simulink model "controller_angular_rate_roll"  (R2020a)
settings: Solver=FixedStepAuto  StartTime=0.0  StopTime=10.0  FixedStep=1/sim_freq  RelTol=1e-3
undefined symbols (not defined in the file): body_rates_dterm_cutoff, body_rates_filter_denom, body_rates_filter_num, d, DiscIntNeverNeededParam, Ixx, K_pd, K_pi, K_pp, max_T, p_int_lim, p_max, tau_T
libraries: simulink x2
settings Model: Creator=francois  LastModifiedBy=murray

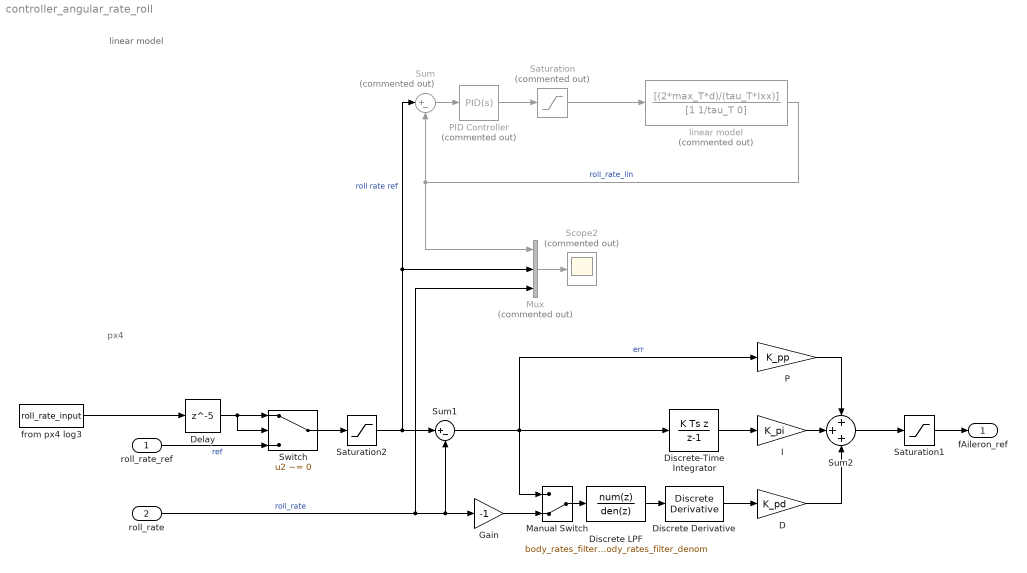
== system controller_angular_rate_roll ==
  note: px4
  note: linear model
  roll_rate_ref : Inport
  roll_rate : Inport  Port=2
  D : Gain  Gain=K_pd
  Delay : Delay  DelayLength=5
  Discrete Derivative : simulink/Discrete/Discrete Derivative  gainval=1.0  ICPrevScaledInput=0.0  OutMin=[]  OutMax=[]  OutDataType=fixdt(1, 16)  OutScaling=2^-10  DoSatur=off
  Discrete LPF : DiscreteTransferFcn  Numerator=body_rates_filter_num  Denominator=body_rates_filter_denom
  Discrete-Time Integrator : DiscreteIntegrator  IntegratorMethod=Integration: Backward Euler  SampleTime=-1  LimitOutput=on  UpperSaturationLimit=p_int_lim  LowerSaturationLimit=-p_int_lim  ICPrevOutput=DiscIntNeverNeededParam  ICPrevScaledInput=DiscIntNeverNeededParam
  Gain : Gain  Gain=-1
  I : Gain  Gain=K_pi
  Manual Switch : ManualSwitch  CurrentSetting=0
  Mux : Mux  Commented=on  Inputs=3
  P : Gain  Gain=K_pp
  "PID Controller " : simulink/Continuous/PID Controller  Commented=on  Controller=PID  Form=Parallel  TimeDomain=Continuous-time  UseExternalTs=off  SampleTime=-1  IntegratorMethod=Forward Euler  FilterMethod=Forward Euler  ControllerParametersSource=internal  P=K_pp  I=K_pi  D=K_pd  UseFilter=on  N=body_rates_dterm_cutoff*10  TunerSelectOption=Transfer Function Based (PID Tuner App)  InitialConditionSource=internal  InitialConditionForIntegrator=0  InitialConditionForFilter=0  DifferentiatorICPrevScaledInput=0  ExternalReset=none  TrackingMode=off  Kt=1  LimitOutput=off  UpperSaturationLimit=inf  LowerSaturationLimit=-inf  LinearizeAsGain=on  AntiWindupMode=none  Kb=1  POutMin=[]  POutMax=[]  IOutMin=[]  IOutMax=[]  DOutMin=[]  DOutMax=[]  NOutMin=[]  NOutMax=[]  SumOutMin=[]  SumOutMax=[]  SaturationOutMin=[]  SaturationOutMax=[]  PParamMin=[]  PParamMax=[]  IParamMin=[]  IParamMax=[]  DParamMin=[]  DParamMax=[]  NParamMin=[]  NParamMax=[]  KbParamMin=[]  KbParamMax=[]  KtParamMin=[]  KtParamMax=[]  KbOutMin=[]  KbOutMax=[]  KtOutMin=[]  KtOutMax=[]  IntegratorOutMin=[]  IntegratorOutMax=[]  FilterOutMin=[]  FilterOutMax=[]  SumI1OutMin=[]  SumI1OutMax=[]  SumI2OutMin=[]  SumI2OutMax=[]  SumI3OutMin=[]  SumI3OutMax=[]  SumI4OutMin=[]  SumI4OutMax=[]  SumDOutMin=[]  SumDOutMax=[]  DifferentiatorOutMin=[]  DifferentiatorOutMax=[]  FilterDiffOutCoefMin=[]  FilterDiffOutCoefMax=[]  ReciprocalOutMin=[]  ReciprocalOutMax=[]  SumDenOutMin=[]  SumDenOutMax=[]  SumNumOutMin=[]  SumNumOutMax=[]  DivideOutMin=[]  DivideOutMax=[]  UdiffTsProdOutMin=[]  UdiffTsProdOutMax=[]  NTsProdOutMin=[]  NTsProdOutMax=[]  UintegralTsProdOutMin=[]  UintegralTsProdOutMax=[]  UngainTsProdOutMin=[]  UngainTsProdOutMax=[]  IntegratorContinuousStateAttributes=''  IntegratorStateMustResolveToSignalObject=off  IntegratorRTWStateStorageClass=Auto  FilterContinuousStateAttributes=''  FilterStateMustResolveToSignalObject=off  FilterRTWStateStorageClass=Auto  ParallelPVariant=InternalParameters  IdealPVariant=Disabled  IVariant=InternalParameters  DVariant=InternalParameters  IntegratorVariant=Continuous  SatVariant=Disabled  AWVariant=Passthrough  PCopyVariant=Disabled  TRVariant=Disabled  FdbkBlocksVariant=Forward  IdealPFdbkVariant=Disabled  SatFdbkVariant=Disabled  DerivativeFilterVariant=ContFilter  NVariant=InternalParameters  NCopyVariant=Disabled  FilterICVariant=InternalICsFilter  IntegratorICVariant=InternalICs  ExternalResetVariant=Disabled  TRSumVariant=Passthrough  SumFdbkVariant=Disabled  SumVariant=Sum_PID  TsampFilterVariant=InternalTs  TsampNgainVariant=Passthrough  TsampIntegralVariant=Passthrough
  Saturation : Saturate  Commented=on  UpperLimit=1  LowerLimit=-1
  Saturation1 : Saturate  UpperLimit=1  LowerLimit=-1
  Saturation2 : Saturate  UpperLimit=p_max  LowerLimit=-p_max
  Scope2 : Scope  Commented=on
  Sum : Sum  Commented=on  Inputs=|+-
  Sum1 : Sum  Inputs=|+-
  Sum2 : Sum  Inputs=+++
  Switch : Switch  Criteria=u2 ~= 0
  from px4 log3 : FromWorkspace  VariableName=roll_rate_input
  linear model : TransferFcn  Commented=on  Numerator=[(2*max_T*d)/(tau_T*Ixx)]  Denominator=[1 1/tau_T 0]
  fAileron_ref : Outport
  wires:
  Sum/1 -> "PID Controller "/1
  roll_rate_ref/1 -> Switch/3  "ref"
  linear model/1 -> Mux/1, Sum/2  "roll_rate_lin"
  Saturation/1 -> linear model/1
  "PID Controller "/1 -> Saturation/1
  Sum1/1 -> Discrete-Time Integrator/1, P/1, Manual Switch/1  "err"
  I/1 -> Sum2/2
  P/1 -> Sum2/1
  D/1 -> Sum2/3
  Discrete-Time Integrator/1 -> I/1
  Discrete Derivative/1 -> D/1
  Manual Switch/1 -> Discrete LPF/1
  Discrete LPF/1 -> Discrete Derivative/1
  Sum2/1 -> Saturation1/1
  Saturation1/1 -> fAileron_ref/1
  roll_rate/1 -> Mux/3, Sum1/2, Gain/1  "roll_rate"
  Gain/1 -> Manual Switch/2
  Saturation2/1 -> Sum1/1, Sum/1, Mux/2  "roll rate ref"
  Switch/1 -> Saturation2/1
  Delay/1 -> Switch/2, Switch/1
  from px4 log3/1 -> Delay/1
  Mux/1 -> Scope2/1
